simulink model "inverted_pendulum_model"  (R2020a)
settings: Solver=VariableStepAuto  StartTime=0.0  StopTime=2  RelTol=1e-3
values from neighbouring files (symbols this model uses):
  b = 0.1    [inverted_pendulum_parameter.m]
  g = 9.8    [inverted_pendulum_parameter.m]
  I = 0.0006    [inverted_pendulum_parameter.m]
  l = 0.3    [inverted_pendulum_parameter.m]
  M = 0.5    [inverted_pendulum_parameter.m]
  m = 0.2    [inverted_pendulum_parameter.m]
libraries: simulink x2
settings Model: Creator=Goku  LastModifiedBy=Goku

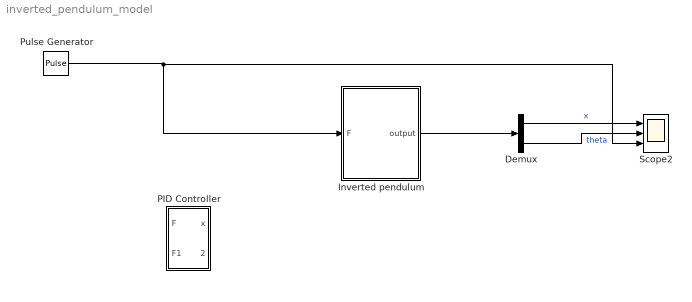
== system inverted_pendulum_model ==
  Demux : Demux  Outputs=2
  Inverted pendulum : Subsystem
  PID Controller : Subsystem
  Pulse Generator : DiscretePulseGenerator  PulseType=Time based  Amplitude=1000  Period=10  PulseWidth=.01
  Scope2 : Scope  NumInputPorts=3
  wires:
  Demux/1 -> Scope2/1  "x"
  Demux/2 -> Scope2/2  "theta"
  Pulse Generator/1 -> Inverted pendulum/1(F), Scope2/3
  Inverted pendulum/1(output) -> Demux/1

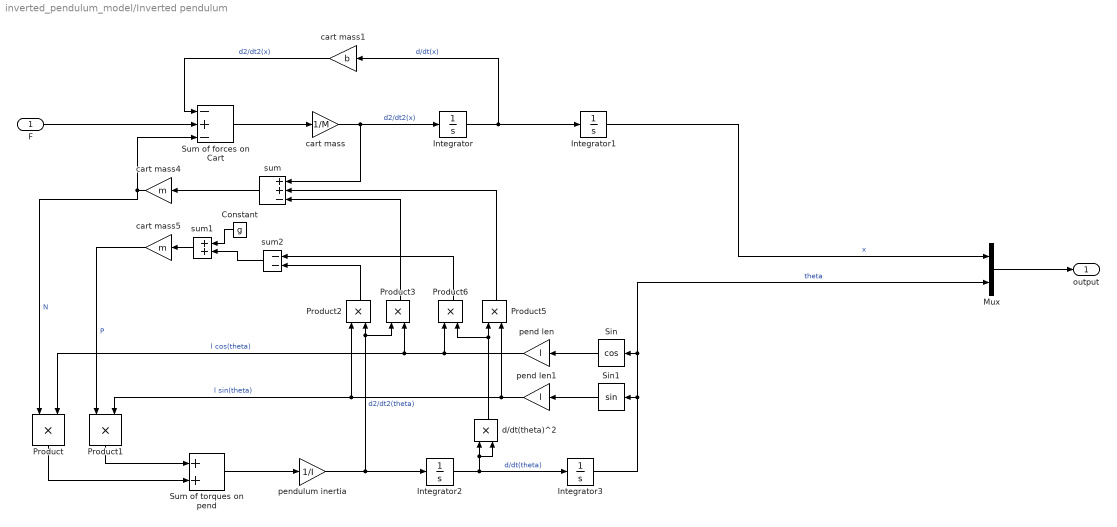
== system inverted_pendulum_model/Inverted pendulum ==
  F : Inport
  Constant : Constant  Value=g
  Integrator{,1..3} (4 alike) : Integrator
  Mux : Mux  Inputs=2
  Product{,1..3,5..6} (6 alike) : Product
  Sin : Trigonometry  Operator=cos
  Sin1 : Trigonometry
  Sum of forces on Cart : Sum  Inputs=-+-
  Sum of torques on pend : Sum
  cart mass : Gain  Gain=1/M
  cart mass1 : Gain  Gain=b
  cart mass4 : Gain  Gain=m
  cart mass5 : Gain  Gain=m
  d/dt(theta)^2 : Product
  pend len : Gain  Gain=l
  pend len1 : Gain  Gain=l
  pendulum inertia : Gain  Gain=1/I
  sum : Sum  Inputs=++-
  sum1 : Sum
  sum2 : Sum  Inputs=--
  output : Outport
  wires:
  Mux/1 -> output/1
  Sum of forces on Cart/1 -> cart mass/1
  Integrator/1 -> cart mass1/1, Integrator1/1  "d/dt(x)"
  Product1/1 -> Sum of torques on pend/1
  Constant/1 -> sum1/1
  Integrator3/1 -> Mux/2, Sin/1, Sin1/1  "theta"
  cart mass5/1 -> Product1/1  "P"
  Product3/1 -> sum/3
  Integrator1/1 -> Mux/1  "x"
  cart mass1/1 -> Sum of forces on Cart/1  "d2/dt2(x)"
  Sin/1 -> pend len/1
  sum2/1 -> sum1/2
  cart mass4/1 -> Product/1, Sum of forces on Cart/3  "N"
  cart mass/1 -> sum/1, Integrator/1  "d2/dt2(x)"
  Sum of torques on pend/1 -> pendulum inertia/1
  Product6/1 -> sum2/1
  pendulum inertia/1 -> Product3/1, Product2/2, Integrator2/1  "d2/dt2(theta)"
  Product/1 -> Sum of torques on pend/2
  F/1 -> Sum of forces on Cart/2
  pend len/1 -> Product6/1, Product3/2, Product/2  "l cos(theta)"
  sum1/1 -> cart mass5/1
  Sin1/1 -> pend len1/1
  Product2/1 -> sum2/2
  d/dt(theta)^2/1 -> Product6/2, Product5/1
  sum/1 -> cart mass4/1
  pend len1/1 -> Product5/2, Product1/2, Product2/1  "l sin(theta)"
  Product5/1 -> sum/2
  Integrator2/1 -> Integrator3/1, d/dt(theta)^2/2, d/dt(theta)^2/1  "d/dt(theta)"

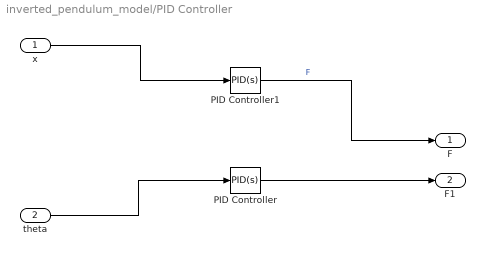
== system inverted_pendulum_model/PID Controller ==
  x : Inport
  theta : Inport  Port=2
  PID Controller : simulink/Continuous/PID Controller  Controller=PID  Form=Parallel  TimeDomain=Continuous-time  UseExternalTs=off  SampleTime=-1  IntegratorMethod=Forward Euler  FilterMethod=Forward Euler  ControllerParametersSource=internal  P=1054.16123700867  I=2212.68658629558  D=61.4720921565294  UseFilter=on  N=100  TunerSelectOption=Transfer Function Based (PID Tuner App)  InitialConditionSource=internal  InitialConditionForIntegrator=0  InitialConditionForFilter=0  DifferentiatorICPrevScaledInput=0  ExternalReset=none  TrackingMode=off  Kt=1  LimitOutput=off  UpperSaturationLimit=inf  LowerSaturationLimit=-inf  LinearizeAsGain=on  AntiWindupMode=none  Kb=1  POutMin=[]  POutMax=[]  IOutMin=[]  IOutMax=[]  DOutMin=[]  DOutMax=[]  NOutMin=[]  NOutMax=[]  SumOutMin=[]  SumOutMax=[]  SaturationOutMin=[]  SaturationOutMax=[]  PParamMin=[]  PParamMax=[]  IParamMin=[]  IParamMax=[]  DParamMin=[]  DParamMax=[]  NParamMin=[]  NParamMax=[]  KbParamMin=[]  KbParamMax=[]  KtParamMin=[]  KtParamMax=[]  KbOutMin=[]  KbOutMax=[]  KtOutMin=[]  KtOutMax=[]  IntegratorOutMin=[]  IntegratorOutMax=[]  FilterOutMin=[]  FilterOutMax=[]  SumI1OutMin=[]  SumI1OutMax=[]  SumI2OutMin=[]  SumI2OutMax=[]  SumI3OutMin=[]  SumI3OutMax=[]  SumI4OutMin=[]  SumI4OutMax=[]  SumDOutMin=[]  SumDOutMax=[]  DifferentiatorOutMin=[]  DifferentiatorOutMax=[]  FilterDiffOutCoefMin=[]  FilterDiffOutCoefMax=[]  ReciprocalOutMin=[]  ReciprocalOutMax=[]  SumDenOutMin=[]  SumDenOutMax=[]  SumNumOutMin=[]  SumNumOutMax=[]  DivideOutMin=[]  DivideOutMax=[]  UdiffTsProdOutMin=[]  UdiffTsProdOutMax=[]  NTsProdOutMin=[]  NTsProdOutMax=[]  UintegralTsProdOutMin=[]  UintegralTsProdOutMax=[]  UngainTsProdOutMin=[]  UngainTsProdOutMax=[]  IntegratorContinuousStateAttributes=''  IntegratorStateMustResolveToSignalObject=off  IntegratorRTWStateStorageClass=Auto  FilterContinuousStateAttributes=''  FilterStateMustResolveToSignalObject=off  FilterRTWStateStorageClass=Auto  ParallelPVariant=InternalParameters  IdealPVariant=Disabled  IVariant=InternalParameters  DVariant=InternalParameters  IntegratorVariant=Continuous  SatVariant=Disabled  AWVariant=Passthrough  PCopyVariant=Disabled  TRVariant=Disabled  FdbkBlocksVariant=Forward  IdealPFdbkVariant=Disabled  SatFdbkVariant=Disabled  DerivativeFilterVariant=ContFilter  NVariant=InternalParameters  NCopyVariant=Disabled  FilterICVariant=InternalICsFilter  IntegratorICVariant=InternalICs  ExternalResetVariant=Disabled  TRSumVariant=Passthrough  SumFdbkVariant=Disabled  SumVariant=Sum_PID  TsampFilterVariant=InternalTs  TsampNgainVariant=Passthrough  TsampIntegralVariant=Passthrough
  PID Controller1 : simulink/Continuous/PID Controller  Controller=PID  Form=Parallel  TimeDomain=Continuous-time  UseExternalTs=off  SampleTime=-1  IntegratorMethod=Forward Euler  FilterMethod=Forward Euler  ControllerParametersSource=internal  P=71849602.5923087  I=33131883567.0561  D=38596.7340197741  UseFilter=on  N=102287.91513606  TunerSelectOption=Transfer Function Based (PID Tuner App)  InitialConditionSource=internal  InitialConditionForIntegrator=0  InitialConditionForFilter=0  DifferentiatorICPrevScaledInput=0  ExternalReset=none  TrackingMode=off  Kt=1  LimitOutput=off  UpperSaturationLimit=inf  LowerSaturationLimit=-inf  LinearizeAsGain=on  AntiWindupMode=none  Kb=1  POutMin=[]  POutMax=[]  IOutMin=[]  IOutMax=[]  DOutMin=[]  DOutMax=[]  NOutMin=[]  NOutMax=[]  SumOutMin=[]  SumOutMax=[]  SaturationOutMin=[]  SaturationOutMax=[]  PParamMin=[]  PParamMax=[]  IParamMin=[]  IParamMax=[]  DParamMin=[]  DParamMax=[]  NParamMin=[]  NParamMax=[]  KbParamMin=[]  KbParamMax=[]  KtParamMin=[]  KtParamMax=[]  KbOutMin=[]  KbOutMax=[]  KtOutMin=[]  KtOutMax=[]  IntegratorOutMin=[]  IntegratorOutMax=[]  FilterOutMin=[]  FilterOutMax=[]  SumI1OutMin=[]  SumI1OutMax=[]  SumI2OutMin=[]  SumI2OutMax=[]  SumI3OutMin=[]  SumI3OutMax=[]  SumI4OutMin=[]  SumI4OutMax=[]  SumDOutMin=[]  SumDOutMax=[]  DifferentiatorOutMin=[]  DifferentiatorOutMax=[]  FilterDiffOutCoefMin=[]  FilterDiffOutCoefMax=[]  ReciprocalOutMin=[]  ReciprocalOutMax=[]  SumDenOutMin=[]  SumDenOutMax=[]  SumNumOutMin=[]  SumNumOutMax=[]  DivideOutMin=[]  DivideOutMax=[]  UdiffTsProdOutMin=[]  UdiffTsProdOutMax=[]  NTsProdOutMin=[]  NTsProdOutMax=[]  UintegralTsProdOutMin=[]  UintegralTsProdOutMax=[]  UngainTsProdOutMin=[]  UngainTsProdOutMax=[]  IntegratorContinuousStateAttributes=''  IntegratorStateMustResolveToSignalObject=off  IntegratorRTWStateStorageClass=Auto  FilterContinuousStateAttributes=''  FilterStateMustResolveToSignalObject=off  FilterRTWStateStorageClass=Auto  ParallelPVariant=InternalParameters  IdealPVariant=Disabled  IVariant=InternalParameters  DVariant=InternalParameters  IntegratorVariant=Continuous  SatVariant=Disabled  AWVariant=Passthrough  PCopyVariant=Disabled  TRVariant=Disabled  FdbkBlocksVariant=Forward  IdealPFdbkVariant=Disabled  SatFdbkVariant=Disabled  DerivativeFilterVariant=ContFilter  NVariant=InternalParameters  NCopyVariant=Disabled  FilterICVariant=InternalICsFilter  IntegratorICVariant=InternalICs  ExternalResetVariant=Disabled  TRSumVariant=Passthrough  SumFdbkVariant=Disabled  SumVariant=Sum_PID  TsampFilterVariant=InternalTs  TsampNgainVariant=Passthrough  TsampIntegralVariant=Passthrough
  F : Outport
  F1 : Outport  Port=2
  wires:
  PID Controller1/1 -> F/1  "F"
  PID Controller/1 -> F1/1
  x/1 -> PID Controller1/1
  theta/1 -> PID Controller/1
